simulink model "TPMS_PlantModel"  (R2025a)
settings: Solver=VariableStepAuto  StartTime=0.0  StopTime=100  RelTol=1e-3
undefined symbols (not defined in the file): C_leak, dPdt_fast, dPdt_slow, P_atm, P_critical, P_initial, P_warn
libraries: fl_lib x6, nesl_utility x3
settings Model: Creator=rauna  LastModifiedBy=rauna
settings ConfigComp: CovEnable=on  RecordCoverage=on  CovModelRefEnable=on

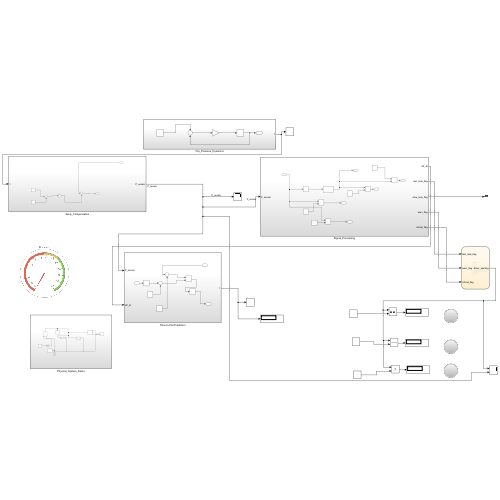
[thumbnail: Simulink's stored preview of the top-level diagram]
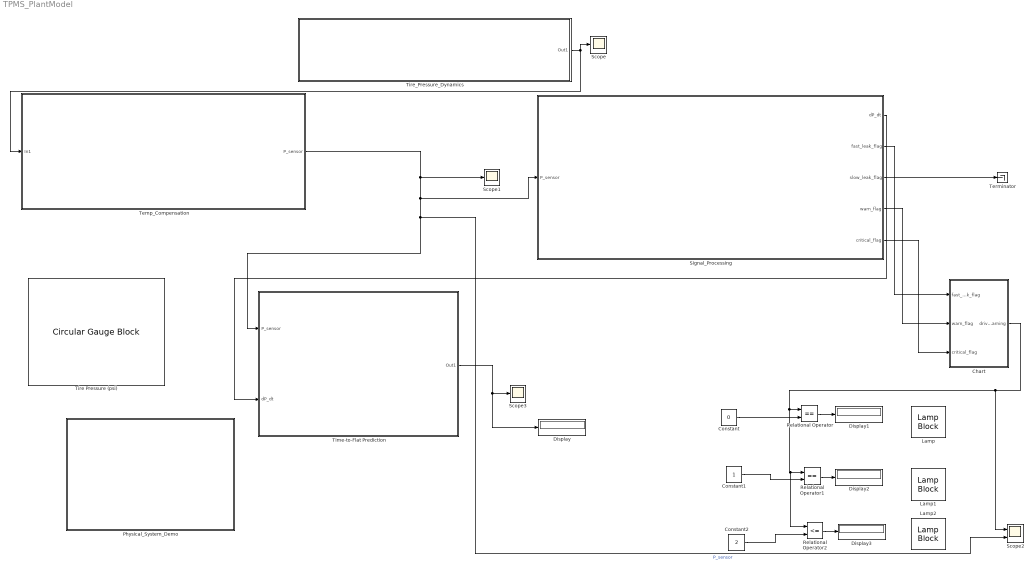
== system TPMS_PlantModel ==
  Chart : Stateflow chart  TreatAsAtomicUnit=on
  Constant : Constant  Value=0
  Constant1 : Constant
  Constant2 : Constant  Value=2
  Display{,1..3} (4 alike) : Display
  Lamp : LampBlock  LabelPosition=Hide  DefaultColor=[192.0, 192.0, 192.0]
  Lamp1 : LampBlock  LabelPosition=Hide  DefaultColor=[192.0, 192.0, 192.0]
  Lamp2 : LampBlock  LabelPosition=Hide  DefaultColor=[192.0, 192.0, 192.0]
  Physical_System_Demo : Subsystem
  Relational Operator : RelationalOperator  Operator===  OutDataTypeStr=boolean  RndMeth=Simplest  InputSameDT=off
  Relational Operator1 : RelationalOperator  Operator===  OutDataTypeStr=boolean  RndMeth=Simplest  InputSameDT=off
  Relational Operator2 : RelationalOperator  Operator=<=  OutDataTypeStr=boolean  RndMeth=Simplest  InputSameDT=off
  Scope : Scope
      settings: ActiveDisplayYMinimum=22.535186861701114  ActiveDisplayYMaximum=51.067685900727682
  Scope1 : Scope
      settings: ActiveDisplayYMinimum=22.891032872693067  ActiveDisplayYMaximum=38.375645456318438
  Scope2 : Scope  NumInputPorts=2
      settings: ActiveDisplayYMinimum=-3.7760795118246939  ActiveDisplayYMaximum=3.6908331328584612  DataLoggingVariableName=ScopeData2
  Scope3 : Scope
      settings: ActiveDisplayYMinimum=-1.1883943434042312  ActiveDisplayYMaximum=2.7342346943615992  DataLoggingVariableName=ScopeData3
  Signal_Processing : Subsystem
  Temp_Compensation : Subsystem
  Terminator : Terminator
  Time-to-Flat Prediction : Subsystem
  Tire Pressure (psi) : CircularGaugeBlock  ScaleMax=40  FontColor=[0.0, 0.0, 0.0]
  Tire_Pressure_Dynamics : Subsystem
  wires:
  Tire_Pressure_Dynamics/1(Out1) -> Scope/1, Temp_Compensation/1(In1)
  Temp_Compensation/1(P_sensor) -> Scope1/1, Scope2/2, Time-to-Flat Prediction/1(P_sensor), Signal_Processing/1(P_sensor)  "P_sensor"
  Signal_Processing/2(fast_leak_flag) -> Chart/1(fast_leak_flag)
  Signal_Processing/4(warn_flag) -> Chart/2(warn_flag)
  Signal_Processing/5(critical_flag) -> Chart/3(critical_flag)
  Time-to-Flat Prediction/1(Out1) -> Display/1, Scope3/1
  Signal_Processing/1(dP_dt) -> Time-to-Flat Prediction/2(dP_dt)
  Signal_Processing/3(slow_leak_flag) -> Terminator/1
  Constant/1 -> Relational Operator/2
  Constant1/1 -> Relational Operator1/2
  Relational Operator/1 -> Display1/1
  Relational Operator1/1 -> Display2/1
  Relational Operator2/1 -> Display3/1
  Chart/1(driver_warning) -> Relational Operator2/1, Relational Operator1/1, Relational Operator/1, Scope2/1
  Constant2/1 -> Relational Operator2/2

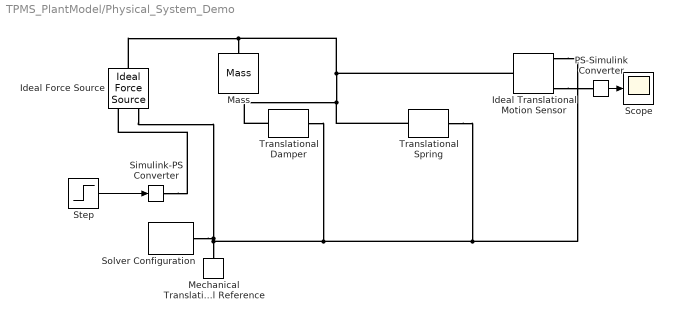
== system TPMS_PlantModel/Physical_System_Demo ==
  Ideal Force Source : fl_lib/Mechanical/Mechanical Sources/Ideal Force Source
  Ideal Translational Motion Sensor : fl_lib/Mechanical/Mechanical Sensors/Ideal Translational Motion Sensor  reference=foundation.enum.MeasurementReference.difference  acceleration_port=false  velocity_port=true  position_port=true  offset=0 m
  Mass : fl_lib/Mechanical/Translational Elements/Mass  mass=1 kg  num_ports=foundation.enum.numPorts2.one  v_specify=off  v_priority=High  v=0 m/s  v_nominal_specify=off  v_nominal_value=1  v_nominal_unit=m/s  f_specify=off  f_priority=None  f=0 N  f_nominal_specify=off  f_nominal_value=1  f_nominal_unit=N
  Mechanical Translational Reference : fl_lib/Mechanical/Translational Elements/Mechanical Translational Reference
  PS-Simulink Converter : nesl_utility/PS-Simulink Converter  PhysicalDomain=network_engine_domain  SubClassName=ps_output  LeftPortType=input  RightPortType=output  PseudoPeriodic=off  Frequencies=[]  VectorFormat=inherit  Unit=inherit  AffineConversion=off
  Scope : Scope
      settings: ActiveDisplayYMinimum=-0.018038348060149811  ActiveDisplayYMaximum=0.16234513254134833  DataLoggingVariableName=ScopeData4
  Simulink-PS Converter : nesl_utility/Simulink-PS Converter  PhysicalDomain=network_engine_domain  SubClassName=ps_input  LeftPortType=input  RightPortType=output  PseudoPeriodic=off  Frequencies=[]  NoiseDistribution=none  NoiseParameters=[]  Unit=1  AffineConversion=off  FilteringAndDerivatives=provide  SimscapeFilterOrder=1  InputFilterTimeConstant=0.001  UdotUserProvided=0
  Solver Configuration : nesl_utility/Solver Configuration  PhysicalDomain=network_engine_domain  SubClassName=solver  LeftPortType=input  RightPortType=generic  Tones=[]  Harmonics=[]  SimulateNoise=off  Profile=off  UseLocalSampling=off  EnableSwitchedLinearOptims=on  FrequencyDomain=off  UseCCode=off  RelTol=0.001  AbsTol=0.001  MinStep=1e-09  ToWorkspace=off  RevertToSquareIcSolve=off  NumHomotopyIterations=100  PhasorMode=off  PhasorModeNumHarmonics=1  ConsistencySolver=NEWTON_XTOL_AFTER_FTOL  IndexReductionMethod=DerivativeReplacement  DoDC=off  ResidualTolerance=1e-09  ConsistencyTolSource=GLOBAL  ConsistencyAbsTol=0.001  ConsistencyRelTol=0.001  ConsistencyTolFactor=0.001  UseLocalSolver=off  LocalSolverChoice=NE_BACKWARD_EULER_ADVANCER  ResolveIndetEquations=on  FunctionEvalNumThread=1  LocalSolverSampleTime=0.001  DoFixedCost=off  MaxNonlinIter=3  MaxModeIter=2  ComputeImpulses=off  ImpulseIterations=2  LinearAlgebra=auto  LinearAlgebraNumThread=0  EquationFormulation=NE_TIME_EF  DelaysMemoryBudget=1024  AutomaticFiltering=on  FilteringTimeConstant=0.001  PartitionStorageMethod=AS_NEEDED  PartitionMemoryBudget=1024  PartitionMethod=ROBUST  MultibodyUseLocalSolver=off  MultibodyLocalSolverChoice=ODE1  MultibodyLocalSolverSampleTime=0.001
  Step : Step  After=10  SampleTime=0
  Translational Damper : fl_lib/Mechanical/Translational Elements/Translational Damper  D=5 N*s/m  v_specify=off  v_priority=None  v=0 m/s  v_nominal_specify=off  v_nominal_value=1  v_nominal_unit=m/s  f_specify=off  f_priority=None  f=0 N  f_nominal_specify=off  f_nominal_value=1  f_nominal_unit=N
  Translational Spring : fl_lib/Mechanical/Translational Elements/Translational Spring  spr_rate=100 N/m  v_specify=off  v_priority=None  v=0 m/s  v_nominal_specify=off  v_nominal_value=1  v_nominal_unit=m/s  f_specify=off  f_priority=None  f=0 N  f_nominal_specify=off  f_nominal_value=1  f_nominal_unit=N  x_specify=off  x_priority=High  x=0 m  x_nominal_specify=off  x_nominal_value=1  x_nominal_unit=m
  wires:
  Step/1 -> Simulink-PS Converter/1
  PS-Simulink Converter/1 -> Scope/1
  connections:
  Ideal Force Source/LConn1 -- Translational Spring/LConn1 -- Translational Damper/LConn1 -- Ideal Translational Motion Sensor/LConn1 -- Mass/LConn1
  Ideal Force Source/RConn2 -- Solver Configuration/RConn1 -- Ideal Translational Motion Sensor/RConn1 -- Translational Spring/RConn1 -- Translational Damper/RConn1 -- Mechanical Translational Reference/LConn1
  Simulink-PS Converter/RConn1 -- Ideal Force Source/RConn1
  Ideal Translational Motion Sensor/RConn3 -- PS-Simulink Converter/LConn1

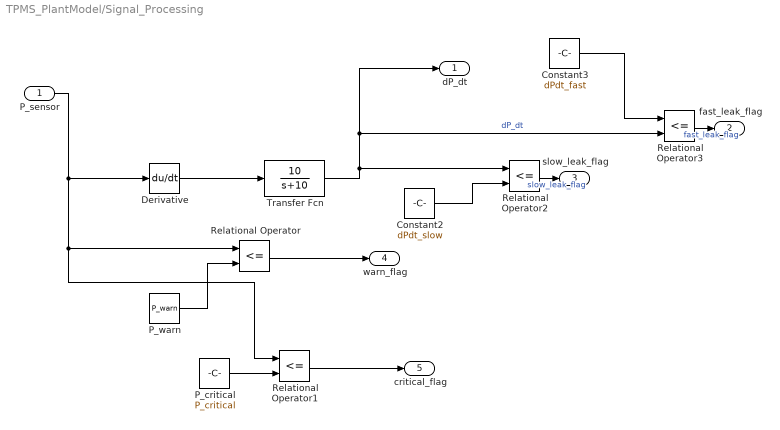
== system TPMS_PlantModel/Signal_Processing ==
  P_sensor : Inport
  Constant2 : Constant  Value=dPdt_slow
  Constant3 : Constant  Value=dPdt_fast
  Derivative : Derivative
  P_critical : Constant  Value=P_critical
  P_warn : Constant  Value=P_warn
  Relational Operator{,1..3} (4 alike) : RelationalOperator  Operator=<=  OutDataTypeStr=boolean  RndMeth=Simplest  InputSameDT=off
  Transfer Fcn : TransferFcn  Numerator=[10]  Denominator=[1 10]
  dP_dt : Outport
  fast_leak_flag : Outport  Port=2
  slow_leak_flag : Outport  Port=3
  warn_flag : Outport  Port=4
  critical_flag : Outport  Port=5
  wires:
  Relational Operator/1 -> warn_flag/1
  Transfer Fcn/1 -> Relational Operator2/1, dP_dt/1, Relational Operator3/2  "dP_dt"
  P_warn/1 -> Relational Operator/2
  Derivative/1 -> Transfer Fcn/1
  Constant3/1 -> Relational Operator3/1
  P_critical/1 -> Relational Operator1/2
  Constant2/1 -> Relational Operator2/2
  Relational Operator1/1 -> critical_flag/1
  P_sensor/1 -> Derivative/1, Relational Operator1/1, Relational Operator/1
  Relational Operator2/1 -> slow_leak_flag/1  "slow_leak_flag"
  Relational Operator3/1 -> fast_leak_flag/1  "fast_leak_flag"

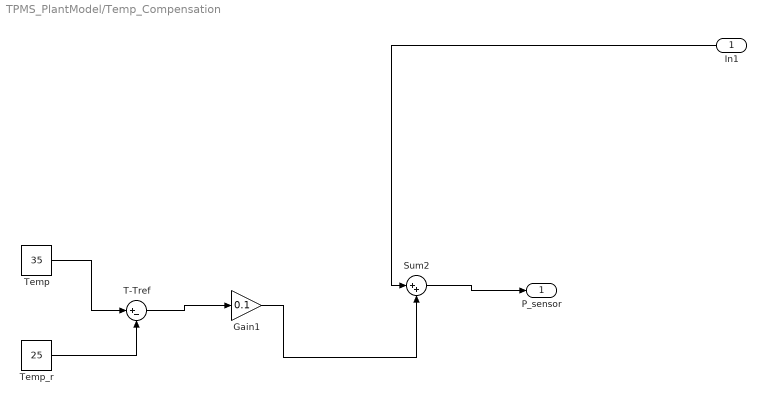
== system TPMS_PlantModel/Temp_Compensation ==
  In1 : Inport
  Gain1 : Gain  Gain=0.1
  Sum2 : Sum  Inputs=|++
  T-Tref : Sum  Inputs=|+-
  Temp : Constant  Value=35
  Temp_r : Constant  Value=25
  P_sensor : Outport
  wires:
  In1/1 -> Sum2/1
  Temp_r/1 -> T-Tref/2
  Sum2/1 -> P_sensor/1
  Temp/1 -> T-Tref/1
  Gain1/1 -> Sum2/2
  T-Tref/1 -> Gain1/1

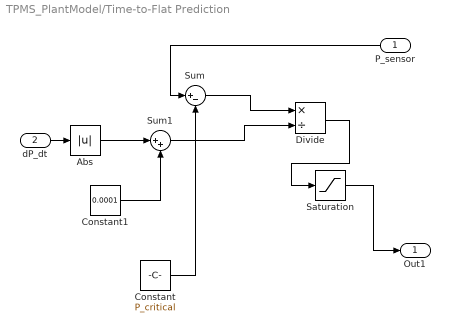
== system TPMS_PlantModel/Time-to-Flat Prediction ==
  P_sensor : Inport
  dP_dt : Inport  Port=2
  Abs : Abs  SaturateOnIntegerOverflow=off
  Constant : Constant  Value=P_critical
  Constant1 : Constant  Value=0.0001
  Divide : Product  Inputs=*/
  Saturation : Saturate
  Sum : Sum  Inputs=|+-
  Sum1 : Sum  Inputs=|++
  Out1 : Outport
  wires:
  Constant/1 -> Sum/2
  Sum/1 -> Divide/1
  Divide/1 -> Saturation/1
  dP_dt/1 -> Abs/1
  Saturation/1 -> Out1/1
  P_sensor/1 -> Sum/1
  Constant1/1 -> Sum1/2
  Abs/1 -> Sum1/1
  Sum1/1 -> Divide/2

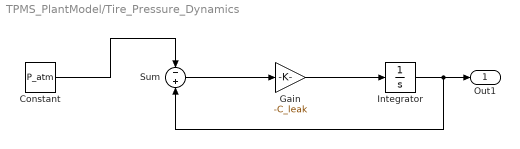
== system TPMS_PlantModel/Tire_Pressure_Dynamics ==
  Constant : Constant  Value=P_atm
  Gain : Gain  Gain=-C_leak
  Integrator : Integrator  InitialCondition=P_initial
  Sum : Sum  Inputs=-+
  Out1 : Outport
  wires:
  Integrator/1 -> Out1/1, Sum/2
  Constant/1 -> Sum/1
  Sum/1 -> Gain/1
  Gain/1 -> Integrator/1

== stateflow chart TPMS_PlantModel/Chart ==
  settings: updateMethod=DISCRETE  sampleTime=1  initializeOutput=1
  state NORMAL
    during: driver_warning = 0;
  state WARNING
    during: driver_warning = 1;
    state SLOW_LEAK
    state FAST_LEAK
    (default) -> SLOW_LEAK
    SLOW_LEAK -> FAST_LEAK : [fast_leak_flag == 1]
    FAST_LEAK -> SLOW_LEAK : [fast_leak_flag == 0]
  state CRITICAL
    during: driver_warning = 2;
  (default) -> NORMAL
  CRITICAL -> NORMAL [order 1] : [critical_flag == 0 && warn_flag == 0]
  NORMAL -> WARNING : [warn_flag == 1]
  WARNING -> NORMAL [order 2] : [warn_flag == 0]
  WARNING -> CRITICAL [order 1] : [critical_flag == 1]
  CRITICAL -> WARNING [order 2] : [critical_flag == 0 && warn_flag == 1]
  data: fast_leak_flag input; warn_flag input; critical_flag input; driver_warning output uint8
